simulink model "pwm_rc_tlv2372_irfp260npbf_simscape"  (R2025a)
settings: Solver=ode23t  StartTime=0.0  StopTime=0.02  MaxStep=1e-6  RelTol=1e-4
libraries: ee_lib x10, fl_lib x6, nesl_utility x6, spiceparts_lib x2
settings Model: Creator=banzang  LastModifiedBy=banzang

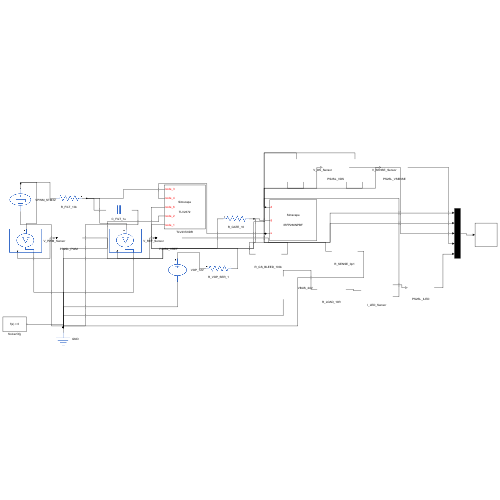
[thumbnail: Simulink's stored preview of the top-level diagram]
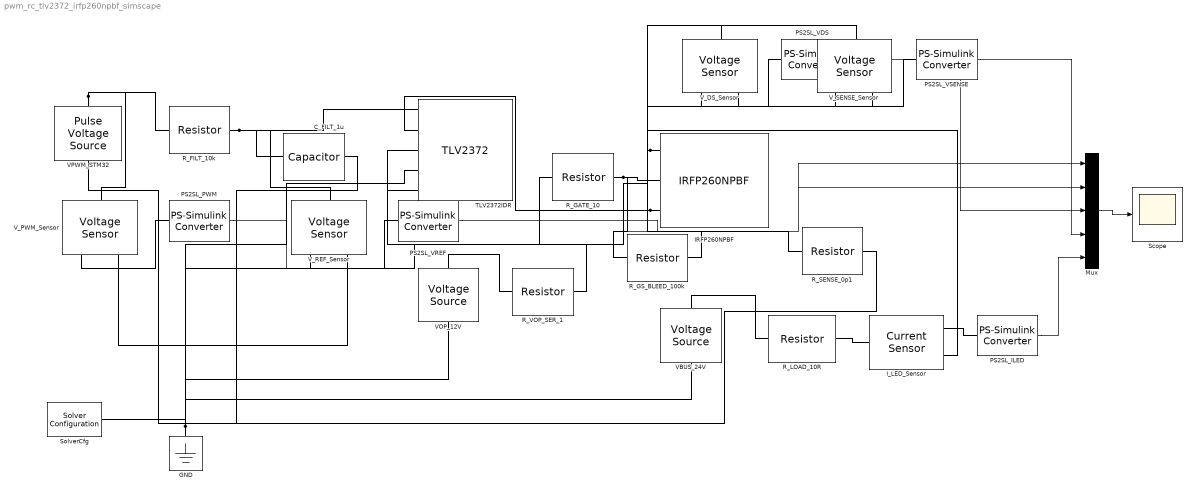
== system pwm_rc_tlv2372_irfp260npbf_simscape ==
  C_FILT_1u : ee_lib/Passive/Capacitor  cap_option=ee.enum.passive.capacitor.capOption.const  c=1e-6 F  Cvec=[1e-05, 1e-06] F  Vvec=[0, 10] V  CV_table_symmetry=ee.enum.passive.capacitor.tableSymmetry.yes  f_vec=[1, 10] kHz  DFext_vec=[.8, 1.2]  enable_C_tol=ee.enum.toleranceApplication.none  averaging_period=0 s  C_tol=5  tol_distribution=ee.enum.toleranceDistribution.uniform  nSigma=4  r=0 Ohm  g=0 1/Ohm  enable_operating_limits=ee.enum.enable.no  operating_limit_action=ee.enum.passive.reportOpLim.warn  max_working_voltage_range=[-25, 25] V  power_rating=1 W  maxTemperature=85 degC  thermalEnable=false  thermalMass=1 J/K  i_specify=off  i_priority=None  i=0 A  i_nominal_specify=off  i_nominal_value=1  i_nominal_unit=A  v_specify=off  v_priority=None  v=0 V  v_nominal_specify=off  v_nominal_value=1  v_nominal_unit=V  vc_specify=off  vc_priority=High  vc=0 V  vc_nominal_specify=off  vc_nominal_value=1  vc_nominal_unit=V  T_specify=off  T_priority=None  T=298.15 K  T_nominal_specify=off  T_nominal_value=1  T_nominal_unit=K
  GND : fl_lib/Electrical/Electrical Elements/Electrical Reference
  IRFP260NPBF : spiceparts_lib/IRFP260NPBF
      settings: InternalSimscapePortConfiguration="{\"Bottom\":[],\"Left\":[{\"id\":\"d\",\"label\":\"d\",\"type\":\"foundation.electrical.electrical\"},{\"id\":\"g\",\"label\":\"g\",\"type\":\"foundation.electrical.electrical\"},{\"id\":\"s\",\"label\":\"s\",\"type\":\"foundation.electrical.electrical\"}],\"Right\":[],\"Top\":[]}"
  I_LED_Sensor : fl_lib/Electrical/Electrical Sensors/Current Sensor
  Mux : Mux  Inputs=5
  PS2SL_ILED : nesl_utility/PS-Simulink Converter  PhysicalDomain=network_engine_domain  SubClassName=ps_output  LeftPortType=input  RightPortType=output  PseudoPeriodic=off  Frequencies=[]  VectorFormat=inherit  Unit=A  AffineConversion=off
  PS2SL_PWM : nesl_utility/PS-Simulink Converter  PhysicalDomain=network_engine_domain  SubClassName=ps_output  LeftPortType=input  RightPortType=output  PseudoPeriodic=off  Frequencies=[]  VectorFormat=inherit  Unit=V  AffineConversion=off
  PS2SL_VDS : nesl_utility/PS-Simulink Converter  PhysicalDomain=network_engine_domain  SubClassName=ps_output  LeftPortType=input  RightPortType=output  PseudoPeriodic=off  Frequencies=[]  VectorFormat=inherit  Unit=V  AffineConversion=off
  PS2SL_VREF : nesl_utility/PS-Simulink Converter  PhysicalDomain=network_engine_domain  SubClassName=ps_output  LeftPortType=input  RightPortType=output  PseudoPeriodic=off  Frequencies=[]  VectorFormat=inherit  Unit=V  AffineConversion=off
  PS2SL_VSENSE : nesl_utility/PS-Simulink Converter  PhysicalDomain=network_engine_domain  SubClassName=ps_output  LeftPortType=input  RightPortType=output  PseudoPeriodic=off  Frequencies=[]  VectorFormat=inherit  Unit=V  AffineConversion=off
  R_FILT_10k : ee_lib/Passive/Resistor  R=10e3 Ohm  enable_R_tol=ee.enum.toleranceApplication.none  R_tol=5  tol_distribution=ee.enum.toleranceDistribution.uniform  nSigma=4  enable_operating_limits=ee.enum.enable.no  operating_limit_action=ee.enum.passive.reportOpLim.warn  power_rating=1 W  max_working_voltage=100 V  noise_mode=ee.enum.sources.noise.Disabled  Tdevice=25 degC  sample_time=1e-3 s  repeatability=ee.enum.ic.repeatability.notRepeatable  user_seed=0  auto_seed=3499211588  power_derating_T1=70 degC  power_derating_T2=155 degC  operating_temperature_range_vec=[-50, 150] degC  alpha=3.93e-3 1/K  Tmeas=25 degC  thermal_mass=100 J/K  temperature_specify=off  temperature_priority=High  temperature=298.15 K  temperature_nominal_specify=off  temperature_nominal_value=1  temperature_nominal_unit=K
  R_GATE_10 : ee_lib/Passive/Resistor  R=10 Ohm  enable_R_tol=ee.enum.toleranceApplication.none  R_tol=5  tol_distribution=ee.enum.toleranceDistribution.uniform  nSigma=4  enable_operating_limits=ee.enum.enable.no  operating_limit_action=ee.enum.passive.reportOpLim.warn  power_rating=1 W  max_working_voltage=100 V  noise_mode=ee.enum.sources.noise.Disabled  Tdevice=25 degC  sample_time=1e-3 s  repeatability=ee.enum.ic.repeatability.notRepeatable  user_seed=0  auto_seed=3890346746  power_derating_T1=70 degC  power_derating_T2=155 degC  operating_temperature_range_vec=[-50, 150] degC  alpha=3.93e-3 1/K  Tmeas=25 degC  thermal_mass=100 J/K  temperature_specify=off  temperature_priority=High  temperature=298.15 K  temperature_nominal_specify=off  temperature_nominal_value=1  temperature_nominal_unit=K
  R_GS_BLEED_100k : ee_lib/Passive/Resistor  R=100e3 Ohm  enable_R_tol=ee.enum.toleranceApplication.none  R_tol=5  tol_distribution=ee.enum.toleranceDistribution.uniform  nSigma=4  enable_operating_limits=ee.enum.enable.no  operating_limit_action=ee.enum.passive.reportOpLim.warn  power_rating=1 W  max_working_voltage=100 V  noise_mode=ee.enum.sources.noise.Disabled  Tdevice=25 degC  sample_time=1e-3 s  repeatability=ee.enum.ic.repeatability.notRepeatable  user_seed=0  auto_seed=545404223  power_derating_T1=70 degC  power_derating_T2=155 degC  operating_temperature_range_vec=[-50, 150] degC  alpha=3.93e-3 1/K  Tmeas=25 degC  thermal_mass=100 J/K  temperature_specify=off  temperature_priority=High  temperature=298.15 K  temperature_nominal_specify=off  temperature_nominal_value=1  temperature_nominal_unit=K
  R_LOAD_10R : ee_lib/Passive/Resistor  R=10 Ohm  enable_R_tol=ee.enum.toleranceApplication.none  R_tol=5  tol_distribution=ee.enum.toleranceDistribution.uniform  nSigma=4  enable_operating_limits=ee.enum.enable.no  operating_limit_action=ee.enum.passive.reportOpLim.warn  power_rating=1 W  max_working_voltage=100 V  noise_mode=ee.enum.sources.noise.Disabled  Tdevice=25 degC  sample_time=1e-3 s  repeatability=ee.enum.ic.repeatability.notRepeatable  user_seed=0  auto_seed=418932850  power_derating_T1=70 degC  power_derating_T2=155 degC  operating_temperature_range_vec=[-50, 150] degC  alpha=3.93e-3 1/K  Tmeas=25 degC  thermal_mass=100 J/K  temperature_specify=off  temperature_priority=High  temperature=298.15 K  temperature_nominal_specify=off  temperature_nominal_value=1  temperature_nominal_unit=K
  R_SENSE_0p1 : ee_lib/Passive/Resistor  R=0.1 Ohm  enable_R_tol=ee.enum.toleranceApplication.none  R_tol=5  tol_distribution=ee.enum.toleranceDistribution.uniform  nSigma=4  enable_operating_limits=ee.enum.enable.no  operating_limit_action=ee.enum.passive.reportOpLim.warn  power_rating=1 W  max_working_voltage=100 V  noise_mode=ee.enum.sources.noise.Disabled  Tdevice=25 degC  sample_time=1e-3 s  repeatability=ee.enum.ic.repeatability.notRepeatable  user_seed=0  auto_seed=3922919431  power_derating_T1=70 degC  power_derating_T2=155 degC  operating_temperature_range_vec=[-50, 150] degC  alpha=3.93e-3 1/K  Tmeas=25 degC  thermal_mass=100 J/K  temperature_specify=off  temperature_priority=High  temperature=298.15 K  temperature_nominal_specify=off  temperature_nominal_value=1  temperature_nominal_unit=K
  R_VOP_SER_1 : ee_lib/Passive/Resistor  R=1 Ohm  enable_R_tol=ee.enum.toleranceApplication.none  R_tol=5  tol_distribution=ee.enum.toleranceDistribution.uniform  nSigma=4  enable_operating_limits=ee.enum.enable.no  operating_limit_action=ee.enum.passive.reportOpLim.warn  power_rating=1 W  max_working_voltage=100 V  noise_mode=ee.enum.sources.noise.Disabled  Tdevice=25 degC  sample_time=1e-3 s  repeatability=ee.enum.ic.repeatability.notRepeatable  user_seed=0  auto_seed=2348838240  power_derating_T1=70 degC  power_derating_T2=155 degC  operating_temperature_range_vec=[-50, 150] degC  alpha=3.93e-3 1/K  Tmeas=25 degC  thermal_mass=100 J/K  temperature_specify=off  temperature_priority=High  temperature=298.15 K  temperature_nominal_specify=off  temperature_nominal_value=1  temperature_nominal_unit=K
  Scope : Scope
  SolverCfg : nesl_utility/Solver Configuration  PhysicalDomain=network_engine_domain  SubClassName=solver  LeftPortType=input  RightPortType=generic  Tones=[]  Harmonics=[]  SimulateNoise=off  Profile=off  UseLocalSampling=off  EnableSwitchedLinearOptims=on  FrequencyDomain=off  UseCCode=off  RelTol=0.001  AbsTol=0.001  MinStep=1e-09  ToWorkspace=off  RevertToSquareIcSolve=off  NumHomotopyIterations=100  PhasorMode=off  PhasorModeNumHarmonics=1  ConsistencySolver=NEWTON_XTOL_AFTER_FTOL  IndexReductionMethod=DerivativeReplacement  DoDC=off  ResidualTolerance=1e-09  ConsistencyTolSource=GLOBAL  ConsistencyAbsTol=0.001  ConsistencyRelTol=0.001  ConsistencyTolFactor=0.001  UseLocalSolver=on  LocalSolverChoice=NE_BACKWARD_EULER_ADVANCER  ResolveIndetEquations=on  FunctionEvalNumThread=1  LocalSolverSampleTime=1e-7  DoFixedCost=off  MaxNonlinIter=3  MaxModeIter=2  ComputeImpulses=off  ImpulseIterations=2  LinearAlgebra=auto  LinearAlgebraNumThread=0  EquationFormulation=NE_TIME_EF  DelaysMemoryBudget=1024  AutomaticFiltering=on  FilteringTimeConstant=0.001  PartitionStorageMethod=AS_NEEDED  PartitionMemoryBudget=1024  PartitionMethod=ROBUST  MultibodyUseLocalSolver=off  MultibodyLocalSolverChoice=ODE1  MultibodyLocalSolverSampleTime=0.001
  TLV2372IDR : spiceparts_lib/TLV2372  specifyParasiticValues=ee.enum.include.yes  capacitorSeriesResistance=1e-3 Ohm  inductorParallelConductance=1e-6 1/Ohm  E2_specify=off  E2_priority=None  E2=0 A  E2_nominal_specify=off  E2_nominal_value=1  E2_nominal_unit=A  E3_specify=off  E3_priority=None  E3=0 A  E3_nominal_specify=off  E3_nominal_value=1  E3_nominal_unit=A  E4_specify=off  E4_priority=None  E4=0 A  E4_nominal_specify=off  E4_nominal_value=1  E4_nominal_unit=A  G2_specify=off  G2_priority=None  G2=0 A  G2_nominal_specify=off  G2_nominal_value=1  G2_nominal_unit=A  E5_specify=off  E5_priority=None  E5=0 A  E5_nominal_specify=off  E5_nominal_value=1  E5_nominal_unit=A  E6_specify=off  E6_priority=None  E6=0 A  E6_nominal_specify=off  E6_nominal_value=1  E6_nominal_unit=A  E7_specify=off  E7_priority=None  E7=0 A  E7_nominal_specify=off  E7_nominal_value=1  E7_nominal_unit=A  E10_specify=off  E10_priority=None  E10=0 A  E10_nominal_specify=off  E10_nominal_value=1  E10_nominal_unit=A  E11_specify=off  E11_priority=None  E11=0 A  E11_nominal_specify=off  E11_nominal_value=1  E11_nominal_unit=A  E12_specify=off  E12_priority=None  E12=0 A  E12_nominal_specify=off  E12_nominal_value=1  E12_nominal_unit=A  E14_specify=off  E14_priority=None  E14=0 A  E14_nominal_specify=off  E14_nominal_value=1  E14_nominal_unit=A  G3_specify=off  G3_priority=None  G3=0 A  G3_nominal_specify=off  G3_nominal_value=1  G3_nominal_unit=A  E17_specify=off  E17_priority=None  E17=0 A  E17_nominal_specify=off  E17_nominal_value=1  E17_nominal_unit=A  E18_specify=off  E18_priority=None  E18=0 A  E18_nominal_specify=off  E18_nominal_value=1  E18_nominal_unit=A  E20_specify=off  E20_priority=None  E20=0 A  E20_nominal_specify=off  E20_nominal_value=1  E20_nominal_unit=A  G7_specify=off  G7_priority=None  G7=0 A  G7_nominal_specify=off  G7_nominal_value=1  G7_nominal_unit=A  G8_specify=off  G8_priority=None  G8=0 A  G8_nominal_specify=off  G8_nominal_value=1  G8_nominal_unit=A  G9_specify=off  G9_priority=None  G9=0 A  G9_nominal_specify=off  G9_nominal_value=1  G9_nominal_unit=A  G10_specify=off  G10_priority=None  G10=0 A  G10_nominal_specify=off  G10_nominal_value=1  G10_nominal_unit=A  E23_specify=off  E23_priority=None  E23=0 A  E23_nominal_specify=off  E23_nominal_value=1  E23_nominal_unit=A  E24_specify=off  E24_priority=None  E24=0 A  E24_nominal_specify=off  E24_nominal_value=1  E24_nominal_unit=A  G11_specify=off  G11_priority=None  G11=0 A  G11_nominal_specify=off  G11_nominal_value=1  G11_nominal_unit=A  G14_specify=off  G14_priority=None  G14=0 A  G14_nominal_specify=off  G14_nominal_value=1  G14_nominal_unit=A  G15_specify=off  G15_priority=None  G15=0 A  G15_nominal_specify=off  G15_nominal_value=1  G15_nominal_unit=A  E48_specify=off  E48_priority=None  E48=0 A  E48_nominal_specify=off  E48_nominal_value=1  E48_nominal_unit=A  E49_specify=off  E49_priority=None  E49=0 A  E49_nominal_specify=off  E49_nominal_value=1  E49_nominal_unit=A  E50_specify=off  E50_priority=None  E50=0 A  E50_nominal_specify=off  E50_nominal_value=1  E50_nominal_unit=A  E94_specify=off  E94_priority=None  E94=0 A  E94_nominal_specify=off  E94_nominal_value=1  E94_nominal_unit=A  G36_specify=off  G36_priority=None  G36=0 A  G36_nominal_specify=off  G36_nominal_value=1  G36_nominal_unit=A  E97_specify=off  E97_priority=None  E97=0 A  E97_nominal_specify=off  E97_nominal_value=1  E97_nominal_unit=A  E98_specify=off  E98_priority=None  E98=0 A  E98_nominal_specify=off  E98_nominal_value=1  E98_nominal_unit=A  E99_specify=off  E99_priority=None  E99=0 A  E99_nominal_specify=off  E99_nominal_value=1  E99_nominal_unit=A  G37_specify=off  G37_priority=None  G37=0 A  G37_nominal_specify=off  G37_nominal_value=1  G37_nominal_unit=A  E100_specify=off  E100_priority=None  E100=0 A  E100_nominal_specify=off  E100_nominal_value=1  E100_nominal_unit=A  G38_specify=off  G38_priority=None  G38=0 A  G38_nominal_specify=off  G38_nominal_value=1  G38_nominal_unit=A
      settings: InternalSimscapePortConfiguration="{\"Bottom\":[],\"Left\":[{\"id\":\"node_3\",\"label\":\"node_3\",\"type\":\"foundation.electrical.electrical\"},{\"id\":\"node_4\",\"label\":\"node_4\",\"type\":\"foundation.electrical.electrical\"},{\"id\":\"node_6\",\"label\":\"node_6\",\"type\":\"foundation.electrical.electrical\"},{\"id\":\"node_2\",\"label\":\"node_2\",\"type\":\"foundation.electrical.electrical\"},{\"id\":\"node_1\",\"label\":\"node_1\",\"type\":\"foundation.electrical.electrical\"}],\"Right\":[],\"Top\":[]}"
  VBUS_24V : ee_lib/Sources/Voltage Source  dc_voltage=24 V  ac_voltage=0 V  ac_shift=0 rad  ac_frequency=60 Hz  noise_mode=ee.enum.sources.noise.Disabled  PSD=0 V^2/Hz  sample_time=1e-3 s  repeatability=ee.enum.sources.repeatability.NotRepeatable  user_seed=0  auto_seed=2715962282  i_specify=off  i_priority=None  i=0 A  i_nominal_specify=off  i_nominal_value=1  i_nominal_unit=A  v_specify=off  v_priority=None  v=0 V  v_nominal_specify=off  v_nominal_value=1  v_nominal_unit=V
  VOP_12V : ee_lib/Sources/Voltage Source  dc_voltage=12 V  ac_voltage=0 V  ac_shift=0 rad  ac_frequency=60 Hz  noise_mode=ee.enum.sources.noise.Disabled  PSD=0 V^2/Hz  sample_time=1e-3 s  repeatability=ee.enum.sources.repeatability.NotRepeatable  user_seed=0  auto_seed=1196140742  i_specify=off  i_priority=None  i=0 A  i_nominal_specify=off  i_nominal_value=1  i_nominal_unit=A  v_specify=off  v_priority=None  v=0 V  v_nominal_specify=off  v_nominal_value=1  v_nominal_unit=V
  VPWM_STM32 : ee_lib/Additional Components/SPICE Sources/Pulse Voltage Source  V1=0 V  V2=3.3 V  TD=2e-3 s  TR=50e-9 s  TF=50e-9 s  PW=1.0e-6 s  PER=20.833e-6 s
      settings: LibrarySourceBlock=ee_lib/Sources/Pulse Voltage Source  InternalSimscapePortConfiguration="{\"Bottom\":[],\"Left\":[{\"id\":\"p\",\"label\":\"\",\"type\":\"foundation.electrical.electrical\"}],\"Right\":[{\"id\":\"n\",\"label\":\"\",\"type\":\"foundation.electrical.electrical\"}],\"Top\":[]}"
  V_DS_Sensor : fl_lib/Electrical/Electrical Sensors/Voltage Sensor
  V_PWM_Sensor : fl_lib/Electrical/Electrical Sensors/Voltage Sensor
  V_REF_Sensor : fl_lib/Electrical/Electrical Sensors/Voltage Sensor
  V_SENSE_Sensor : fl_lib/Electrical/Electrical Sensors/Voltage Sensor
  wires:
  PS2SL_PWM/1 -> Mux/1
  PS2SL_VREF/1 -> Mux/2
  PS2SL_VDS/1 -> Mux/3
  PS2SL_VSENSE/1 -> Mux/4
  PS2SL_ILED/1 -> Mux/5
  Mux/1 -> Scope/1
  connections:
  SolverCfg/RConn1 -- VPWM_STM32/RConn1 -- VBUS_24V/RConn1 -- VOP_12V/RConn1 -- C_FILT_1u/RConn1 -- TLV2372IDR/LConn4 -- R_SENSE_0p1/RConn1 -- V_PWM_Sensor/RConn2 -- V_REF_Sensor/RConn2 -- GND/LConn1 -- V_SENSE_Sensor/RConn2
  R_FILT_10k/LConn1 -- VPWM_STM32/LConn1 -- V_PWM_Sensor/LConn1
  C_FILT_1u/LConn1 -- R_FILT_10k/RConn1 -- TLV2372IDR/LConn1 -- V_REF_Sensor/LConn1
  VOP_12V/LConn1 -- R_VOP_SER_1/LConn1
  R_VOP_SER_1/RConn1 -- TLV2372IDR/LConn3
  TLV2372IDR/LConn5 -- R_GATE_10/LConn1
  IRFP260NPBF/LConn2 -- R_GATE_10/RConn1 -- R_GS_BLEED_100k/LConn1
  R_GS_BLEED_100k/RConn1 -- R_SENSE_0p1/LConn1 -- TLV2372IDR/LConn2 -- V_DS_Sensor/RConn2 -- IRFP260NPBF/LConn3 -- V_SENSE_Sensor/LConn1
  VBUS_24V/LConn1 -- R_LOAD_10R/LConn1
  R_LOAD_10R/RConn1 -- I_LED_Sensor/LConn1
  IRFP260NPBF/LConn1 -- I_LED_Sensor/RConn2 -- V_DS_Sensor/LConn1
  V_PWM_Sensor/RConn1 -- PS2SL_PWM/LConn1
  V_REF_Sensor/RConn1 -- PS2SL_VREF/LConn1
  V_DS_Sensor/RConn1 -- PS2SL_VDS/LConn1
  V_SENSE_Sensor/RConn1 -- PS2SL_VSENSE/LConn1
  I_LED_Sensor/RConn1 -- PS2SL_ILED/LConn1
